simulink model "controlsystem"  (R2017a)
settings: Solver=VariableStepAuto  StartTime=0.0  StopTime=10.0  RelTol=1e-3
settings Model: Creator=Jash  LastModifiedBy=Jash

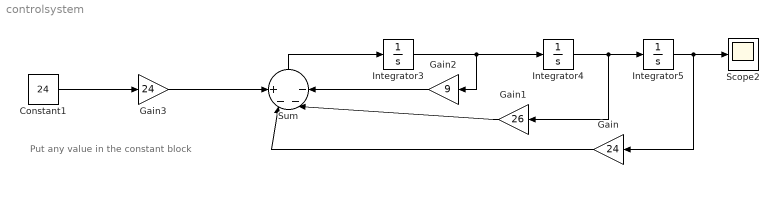
== system controlsystem ==
  note: Put any value in the constant block
  Constant1 : Constant  Value=24
  Gain : Gain  Gain=24
  Gain1 : Gain  Gain=26
  Gain2 : Gain  Gain=9
  Gain3 : Gain  Gain=24
  Integrator3 : Integrator
  Integrator4 : Integrator
  Integrator5 : Integrator
  Scope2 : Scope
  Sum : Sum  Inputs=+|-|-|-
  wires:
  Constant1/1 -> Gain3/1
  Gain3/1 -> Sum/1
  Sum/1 -> Integrator3/1
  Gain/1 -> Sum/2
  Gain1/1 -> Sum/3
  Gain2/1 -> Sum/4
  Integrator3/1 -> Gain2/1, Integrator4/1
  Integrator5/1 -> Scope2/1, Gain/1
  Integrator4/1 -> Integrator5/1, Gain1/1
